simulink model "uloha1_sim"  (R2014a)
settings: Solver=ode3  StartTime=0.0  StopTime=10  FixedStep=.1  RelTol=1e-6
values from neighbouring files (symbols this model uses):
  B = selbest(POP,I,ones(1,13))    [AAACviko_05.m]    (also in crit_fun2.m = 0.01; uloha1.m = 0.01)
  b = B    (= 0.01)    [crit_fun2.m]    (also in uloha1.m)
  g = 9.81    [crit_fun2.m]    (also in uloha1.m)
  J = m*l^2    (= 0.032)    [crit_fun2.m]    (also in uloha1.m)
  K = -1/g    (= -0.101936799185)    [crit_fun2.m]    (also in uloha1.m)
  Kd = Najlepsi_vysledok(3)    [AAACviko_05.m]    (also in crit_fun.m = POP(i,3); crit_fun2.m = POP(i,3))
  Kp = Najlepsi_vysledok(1)    [AAACviko_05.m]    (also in crit_fun.m = POP(i,1); crit_fun2.m = POP(i,1))
  l = 0.4    [crit_fun2.m]    (also in uloha1.m)
  m = 0.2    [crit_fun2.m]    (also in gennumbers.m = 10; uloha1.m)
  w = sqrt(g/l)    [crit_fun2.m]    (also in uloha1.m)
settings Model: Creator=Michal  LastModifiedBy=tomas
settings DebuggingCC: MergeDetectMultiDrivingBlocksExec=error

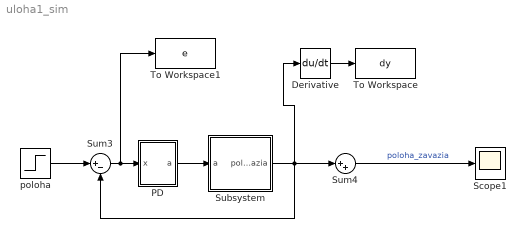
== system uloha1_sim ==
  Derivative : Derivative
  PD : Subsystem
  Scope1 : Scope
  Subsystem : Subsystem
      mask Display: disp('zavazie')
  Sum3 : Sum  Inputs=|+-
  Sum4 : Sum  Inputs=|++
  To Workspace : ToWorkspace  VariableName=dy  SampleTime=-1
  To Workspace1 : ToWorkspace  VariableName=e  SampleTime=-1
  poloha : Step  Time=0  SampleTime=0
  wires:
  poloha/1 -> Sum3/1
  Sum3/1 -> To Workspace1/1, PD/1(x)
  Sum4/1 -> Scope1/1  "poloha_zavazia"
  PD/1(a) -> Subsystem/1(a)
  Subsystem/1(poloha zavazia) -> Derivative/1, Sum4/1, Sum3/2
  Derivative/1 -> To Workspace/1

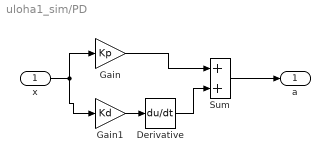
== system uloha1_sim/PD ==
  x : Inport
  Derivative : Derivative
  Gain : Gain  Gain=Kp
  Gain1 : Gain  Gain=Kd
  Sum : Sum
  a : Outport
  wires:
  Gain/1 -> Sum/1
  Derivative/1 -> Sum/2
  Gain1/1 -> Derivative/1
  x/1 -> Gain1/1, Gain/1
  Sum/1 -> a/1

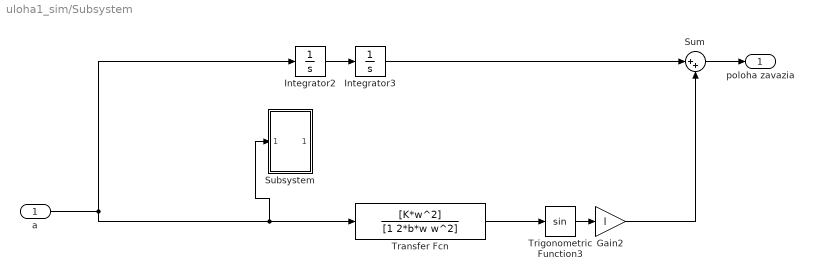
== system uloha1_sim/Subsystem ==
  a : Inport
  Gain2 : Gain  Gain=l
  Integrator2 : Integrator
  Integrator3 : Integrator
  Subsystem : Subsystem
  Sum : Sum  Inputs=|++
  Transfer Fcn : TransferFcn  Numerator=[K*w^2]  Denominator=[1 2*b*w w^2]
  Trigonometric Function3 : Trigonometry
  poloha zavazia : Outport
  wires:
  a/1 -> Transfer Fcn/1, Subsystem/1(In1), Integrator2/1
  Integrator2/1 -> Integrator3/1
  Integrator3/1 -> Sum/1
  Sum/1 -> poloha zavazia/1
  Transfer Fcn/1 -> Trigonometric Function3/1
  Trigonometric Function3/1 -> Gain2/1
  Gain2/1 -> Sum/2

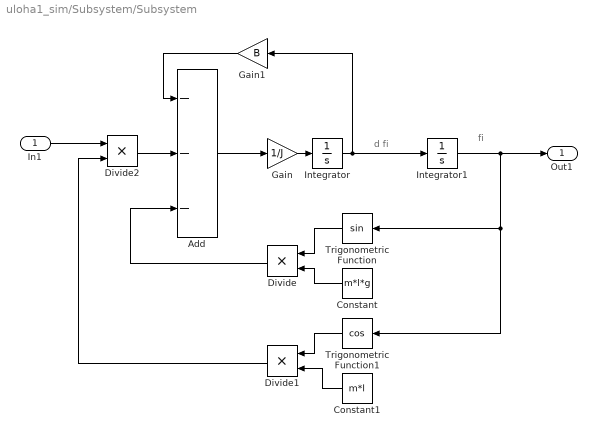
== system uloha1_sim/Subsystem/Subsystem ==
  note: fi
  note: d fi
  In1 : Inport
  Add : Sum  Inputs=---
  Constant : Constant  Value=m*l*g
  Constant1 : Constant  Value=m*l
  Divide : Product  Inputs=**
  Divide1 : Product  Inputs=**
  Divide2 : Product  Inputs=**
  Gain : Gain  Gain=1/J
  Gain1 : Gain  Gain=B
  Integrator : Integrator
  Integrator1 : Integrator
  Trigonometric Function : Trigonometry
  Trigonometric Function1 : Trigonometry  Operator=cos
  Out1 : Outport
  wires:
  Integrator/1 -> Gain1/1, Integrator1/1
  Add/1 -> Gain/1
  Trigonometric Function1/1 -> Divide1/1
  Constant/1 -> Divide/2
  Gain/1 -> Integrator/1
  Trigonometric Function/1 -> Divide/1
  Constant1/1 -> Divide1/2
  Divide/1 -> Add/3
  Gain1/1 -> Add/1
  Integrator1/1 -> Out1/1, Trigonometric Function1/1, Trigonometric Function/1
  Divide2/1 -> Add/2
  Divide1/1 -> Divide2/2
  In1/1 -> Divide2/1
